simulink model "pwctrl"  (Simulink 7.8)
settings: Solver=FixedStepDiscrete  StartTime=0.0  StopTime=10  FixedStep=Ts  RelTol=1e-2
values from neighbouring files (symbols this model uses):
  EndStopThreshold = 15    [pwctrl_data.m]
  ObstacleThreshold = 1.2    [pwctrl_data.m]
undefined symbols (not defined in the file or in its folder): gcbh, rmidispblock
settings Model: RequirementInfo={'doors' '0000006a' '1' 'false' 'DOORS Surrogate Item' '' } %GIDa_dde32420_d5f5_4b5c_860d_5475e0ff803b  reqMgrSettings="100 S'doors','misc'{{S'surrogatepath','savemodel','savesurrogate','updateLinks','doorsLinks2sl','slLinks2Doors','purgeDoors','purgeSimulink','detaillevel','surrogateId','synctime'{{T\"/PowerWindow/pwctrl\",M[1],M[1],M[1],M[0],M[1],M[0],M[0],M[1],T\"0000006a\",T\"\"}},S'mode','pathStorage'{{T\"generic\",T\"modelRelative\"}}}}"  Creator=The MathWorks Inc.  LastModifiedBy=itoy  CovSaveName=covdatac  CovMetricSettings=dcmw  CovHTMLOptions=-aTS=1 -bRG=1 -bTC=1 -hTR=0 -nFC=0 -scm=1 -bcm=1 -xEv=0  CovCumulativeVarName=covCumulativeDataPwctrl  ExtModeAutoUpdateStatusClock=off
settings DataIOCC: SaveOutput=off  SaveTime=off  SignalLoggingName=sigsOut
settings OptimizationCC: InlineParams=on  InlineInvariantSignals=on  InitFltsAndDblsToZero=on  OptimizeModelRefInitCode=on  LifeSpan=1
settings DebuggingCC: SignalInfNanChecking=error  SaveWithParameterizedLinksMsg=none  CheckExecutionContextPreStartOutputMsg=on  CheckExecutionContextRuntimeOutputMsg=on  SolverPrmCheckMsg=none  MultiTaskDSMMsg=warning  MultiTaskCondExecSysMsg=none  ParameterUnderflowMsg=error  ParameterPrecisionLossMsg=error  ParameterTunabilityLossMsg=error  FcnCallInpInsideContextMsg=Use local settings  UniqueDataStoreMsg=warning  BusObjectLabelMismatch=error  RootOutportRequireBusObject=error  BusNameAdapt=ErrorWithoutRepair  NonBusSignalsTreatedAsBus=error
settings HardwareCC: ProdHWDeviceType=Generic->Unspecified (assume 32-bit Generic)  TargetIntDivRoundTo=Zero  TargetEndianess=LittleEndian  TargetHWDeviceType=Generic->MATLAB Host Computer  ProdEqTarget=off
settings SFSimCC: SimParseCustomCode=off
settings RTWCC: SystemTargetFile=ert.tlc  GenCodeOnly=on  TemplateMakefile=ert_default_tmf  Description=Real-Time Workshop Embedded Coder  GenerateReport=on  ProcessScript=ert_make_rtw_hook  IncludeHyperlinkInReport=on  LaunchReport=on  IncludeERTFirstTime=on  GenerateTraceInfo=on  GenerateTraceReport=on  GenerateTraceReportSl=on  GenerateTraceReportSf=on  GenerateTraceReportEml=on  GenerateCodeMetricsReport=on
settings MATStruct: className=rtw.pil.Bullseye  argsAllComponents=[]  excludedModels=[]  includeReferencedModels=off  includeTopModel=on  enabled=off
settings CodeAppCC: IgnoreCustomStorageClasses=off  CustomSymbolStrFcn=$F$N$M  ReqsInCode=on
settings ERTTargetCC: MultiwordLength=2048  GenerateSampleERTMain=on  SupportAbsoluteTime=off  SupportComplex=off  InlinedParameterPlacement=NonHierarchical  ERTCustomFileTemplate=example_file_process.tlc  ConvertIfToSwitch=off  SuppressUnreachableDefaultCases=off
settings SimMechanicsCC: WarnOnRedundantConstraints=off  VisOnUpdateDiagram=on
settings ConfigComp: Description=Design Verifier Custom Configuration Component  DVMaxProcessTime=600  DVDisplayUnsatisfiableObjectives=on  DVAutomaticStubbing=off  DVParametersConfigFileName=pwctrl_sldvparam.m  DVModelCoverageObjectives=MCDC  DVMaxTestCaseSteps=500  DVTestSuiteOptimization=CombinedObjectives (Nonlinear Extended)  DVIgnoreExistTestSatisfied=off  DVCoverageDataFile=C:\work\EXPO2010\demo\topmodelCov.cvt  DVSaveHarnessModel=on  DVSaveReport=on  DVDisplayResultsOnModel=on

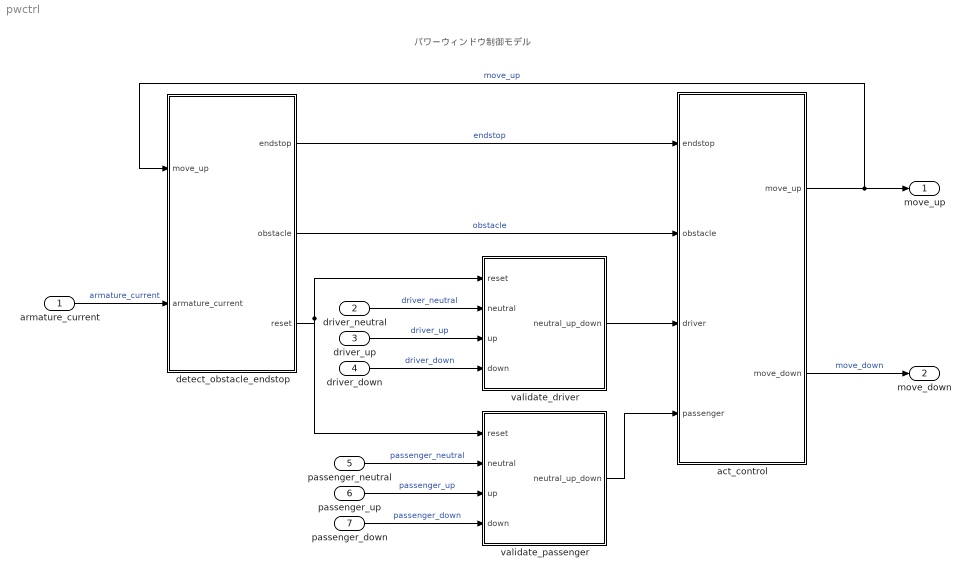
== system pwctrl ==
  note: パワーウィンドウ制御モデル
  armature_current : Inport  RequirementInfo={'other' 'powerwindowspecification.xlsx' '@Simulink_requirement_item_1' 'true' '電機子電流' '' } %GIDa_e1c18c69_aba9_407e_934a_76d29523162c  OutDataTypeStr=double  PortDimensions=1  Interpolate=off
  driver_neutral : Inport  RequirementInfo={'other' 'powerwindowspecification.xlsx' '@Simulink_requirement_item_2' 'true' '運転席ニュートラル命令' '' ; 'other' 'テスト01.docx' '@Simulink_requirement_item_1' 'true' 'テスト01' '' } %GIDa_63218ceb_c29f_4eb9_95a6_9012dd0a3532  Port=2  OutDataTypeStr=boolean  PortDimensions=1  Interpolate=off
  driver_up : Inport  RequirementInfo={'other' 'powerwindowspecification.xlsx' '@Simulink_requirement_item_3' 'true' '運転席アップ命令' '' } %GIDa_0b230fa1_5c49_495f_8d06_8dd23c30b7f9  Port=3  OutDataTypeStr=boolean  PortDimensions=1  Interpolate=off
  driver_down : Inport  RequirementInfo={'other' 'powerwindowspecification.xlsx' '@Simulink_requirement_item_4' 'true' '運転席ダウン命令' '' } %GIDa_6ce8d57e_d33e_47fb_aa6f_8cf7e75a9f12  Port=4  OutDataTypeStr=boolean  PortDimensions=1  Interpolate=off
  passenger_neutral : Inport  RequirementInfo={'other' 'powerwindowspecification.xlsx' '@Simulink_requirement_item_5' 'true' '助手席ニュートラル命令' '' } %GIDa_26eb5b41_6f4f_4623_9fef_cd17cf2cf6e8  Port=5  OutDataTypeStr=boolean  PortDimensions=1  Interpolate=off
  passenger_up : Inport  RequirementInfo={'other' 'powerwindowspecification.xlsx' '@Simulink_requirement_item_6' 'true' '助手席アップ命令' '' } %GIDa_f768338e_5d08_4c2e_8a73_e293dd283a19  Port=6  OutDataTypeStr=boolean  PortDimensions=1  Interpolate=off
  passenger_down : Inport  RequirementInfo={'other' 'powerwindowspecification.xlsx' '@Simulink_requirement_item_7' 'true' '助手席ダウン命令' '' } %GIDa_640f9234_8c00_498e_835c_04d6c270f85b  Port=7  OutDataTypeStr=boolean  PortDimensions=1  Interpolate=off
  act_control : Stateflow chart  RequirementInfo="{}  %GIDa_ef77f4d8_d6ef_4c80_8fd6_c4e6f18a1482"  TreatAsAtomicUnit=on
  detect_obstacle_endstop : Subsystem  RequirementInfo={'other' 'powerwindowspecification.xlsx' '@Simulink_requirement_item_75' 'true' 'PW02 障害物検知' '' ; 'other' 'powerwindowspecification.xlsx' '@Simulink_requirement_item_76' 'true' 'PW01-6' '' } %GIDa_a872e992_2f76_4f1e_be0d_48f835553ea8  TreatAsAtomicUnit=on
  validate_driver : Subsystem  RequirementInfo={'other' 'powerwindowspecification.xlsx' '@Simulink_requirement_item_74' 'true' 'PW01-1' '' ; 'other' 'powerwindowspecification.xlsx' '@Simulink_requirement_item_11' 'true' 'PW01-2' '' ; 'other' 'powerwindowspecification.xlsx' '@Simulink_requirement_item_12' 'true' 'PW01-3' '' } %GIDa_50d6339c_d923_4cb4_be9a_59dfda00bcf8  TreatAsAtomicUnit=on
  validate_passenger : Subsystem  RequirementInfo={'other' 'powerwindowspecification.xlsx' '@Simulink_requirement_item_13' 'true' 'PW01-4' '' ; 'other' 'powerwindowspecification.xlsx' '@Simulink_requirement_item_14' 'true' 'PW01-5' '' ; 'other' 'powerwindowspecification.xlsx' '@Simulink_requirement_item_15' 'true' 'PW01-6' '' } %GIDa_266d8f5a_6cdb_435d_b6a4_e11a48d16765  TreatAsAtomicUnit=on
  move_up : Outport  RequirementInfo={'other' 'powerwindowspecification.xlsx' '@Simulink_requirement_item_8' 'true' 'アップ指示' '' } %GIDa_af57c1a9_bee2_4bf2_aa23_d9548663e543  OutDataTypeStr=boolean
  move_down : Outport  RequirementInfo={'other' 'powerwindowspecification.xlsx' '@Simulink_requirement_item_9' 'true' 'ダウン指示' '' } %GIDa_5b47727d_3f56_4ff6_a9b6_2b328d3a62d1  Port=2  OutDataTypeStr=boolean
  wires:
  validate_passenger/1(neutral_up_down) -> act_control/4(passenger)
  validate_driver/1(neutral_up_down) -> act_control/3(driver)
  passenger_down/1 -> validate_passenger/4(down)  "passenger_down"
  passenger_up/1 -> validate_passenger/3(up)  "passenger_up"
  passenger_neutral/1 -> validate_passenger/2(neutral)  "passenger_neutral"
  driver_down/1 -> validate_driver/4(down)  "driver_down"
  driver_up/1 -> validate_driver/3(up)  "driver_up"
  driver_neutral/1 -> validate_driver/2(neutral)  "driver_neutral"
  act_control/2(move_down) -> move_down/1  "move_down"
  act_control/1(move_up) -> move_up/1, detect_obstacle_endstop/1(move_up)  "move_up"
  armature_current/1 -> detect_obstacle_endstop/2(armature_current)  "armature_current"
  detect_obstacle_endstop/3(reset) -> validate_driver/1(reset), validate_passenger/1(reset)
  detect_obstacle_endstop/1(endstop) -> act_control/1(endstop)  "endstop"
  detect_obstacle_endstop/2(obstacle) -> act_control/2(obstacle)  "obstacle"

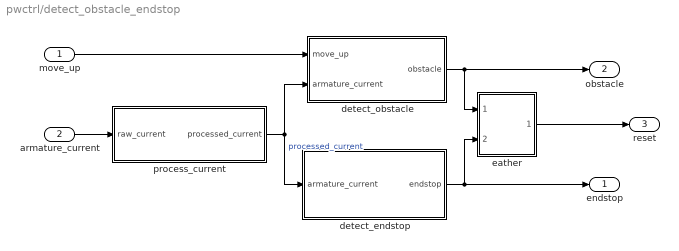
== system pwctrl/detect_obstacle_endstop ==
  move_up : Inport
  armature_current : Inport  Port=2
  detect_endstop : Subsystem  RequirementInfo={'other' 'powerwindowspecification.xlsx' '@Simulink_requirement_item_41' 'true' 'PW03-1' '' } %GIDa_aaa80572_f933_4bbe_b37f_c57c83952132
  detect_obstacle : Subsystem  RequirementInfo={'other' 'powerwindowspecification.xlsx' '@Simulink_requirement_item_33' 'true' 'PW02-1' '' } %GIDa_e14b3a63_7ae7_416e_9be9_c6135a02f311
  eather : Subsystem
  process_current : Subsystem  RequirementInfo={'other' 'powerwindowspecification.xlsx' '@Simulink_requirement_item_32' 'true' 'PW02-1' '' ; 'other' 'powerwindowspecification.xlsx' '@Simulink_requirement_item_40' 'true' 'PW03-1' '' } %GIDa_54e86e3e_ccc8_4b41_a5c1_edc4e8429aa2
  endstop : Outport
  obstacle : Outport  Port=2
  reset : Outport  Port=3
  wires:
  process_current/1(processed_current) -> detect_endstop/1(armature_current), detect_obstacle/2(armature_current)  "processed_current"
  move_up/1 -> detect_obstacle/1(move_up)
  eather/1(reset) -> reset/1
  detect_endstop/1(endstop) -> eather/2(endstop), endstop/1
  detect_obstacle/1(obstacle) -> obstacle/1, eather/1(obstacle)
  armature_current/1 -> process_current/1(raw_current)

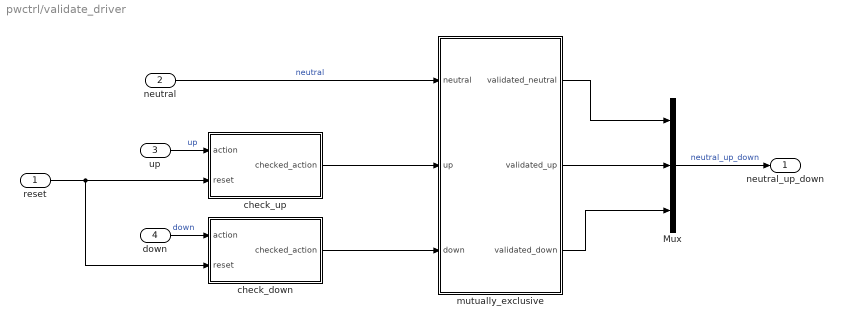
== system pwctrl/validate_driver ==
  reset : Inport
  neutral : Inport  Port=2
  up : Inport  Port=3
  down : Inport  Port=4
  Mux : Mux  Inputs=3
  check_down : Subsystem  RequirementInfo={'other' 'powerwindowspecification.xlsx' '@Simulink_requirement_item_55' 'true' 'PW02-4' '' ; 'other' 'powerwindowspecification.xlsx' '@Simulink_requirement_item_48' 'true' 'PW03-3' '' } %GIDa_8600958e_cd26_4390_bd74_0e0e2b2911b6
  check_up : Subsystem  RequirementInfo={'other' 'powerwindowspecification.xlsx' '@Simulink_requirement_item_54' 'true' 'PW02-4' '' ; 'other' 'powerwindowspecification.xlsx' '@Simulink_requirement_item_47' 'true' 'PW03-3' '' } %GIDa_854a0f09_eb00_4639_b606_a3908bff6a10
  mutually_exclusive : Subsystem  RequirementInfo={'other' 'powerwindowspecification.xlsx' '@Simulink_requirement_item_26' 'true' 'PW01-2-3' '' ; 'other' 'powerwindowspecification.xlsx' '@Simulink_requirement_item_29' 'true' 'PW01-1-3' '' } %GIDa_ad342d9f_5cab_43fb_a439_1578864a89a4
  neutral_up_down : Outport
  wires:
  Mux/1 -> neutral_up_down/1  "neutral_up_down"
  reset/1 -> check_down/2(reset), check_up/2(reset)
  check_up/1(checked_action) -> mutually_exclusive/2(up)
  neutral/1 -> mutually_exclusive/1(neutral)  "neutral"
  up/1 -> check_up/1(action)  "up"
  down/1 -> check_down/1(action)  "down"
  mutually_exclusive/1(validated_neutral) -> Mux/1
  mutually_exclusive/2(validated_up) -> Mux/2
  mutually_exclusive/3(validated_down) -> Mux/3
  check_down/1(checked_action) -> mutually_exclusive/3(down)

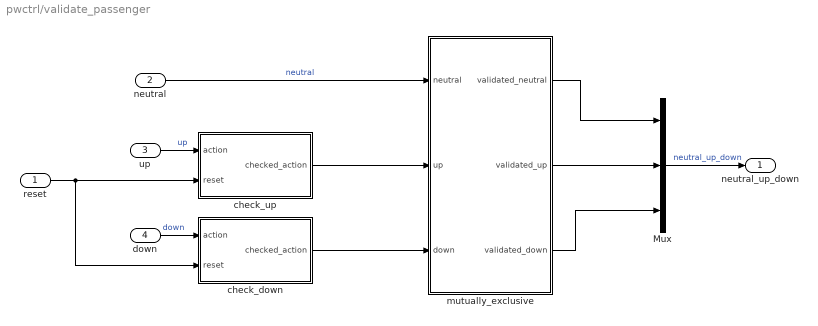
== system pwctrl/validate_passenger ==
  reset : Inport
  neutral : Inport  Port=2
  up : Inport  Port=3
  down : Inport  Port=4
  Mux : Mux  Inputs=3
  check_down : Subsystem  RequirementInfo={'other' 'powerwindowspecification.xlsx' '@Simulink_requirement_item_53' 'true' 'PW02-4' '' ; 'other' 'powerwindowspecification.xlsx' '@Simulink_requirement_item_50' 'true' 'PW03-3' '' } %GIDa_be4e89e9_75a8_4fb1_9b06_a19403e0c6cf
  check_up : Subsystem  RequirementInfo={'other' 'powerwindowspecification.xlsx' '@Simulink_requirement_item_52' 'true' 'PW02-4' '' ; 'other' 'powerwindowspecification.xlsx' '@Simulink_requirement_item_49' 'true' 'PW03-3' '' } %GIDa_c1637765_e427_4142_80f6_8167853f7876
  mutually_exclusive : Subsystem  RequirementInfo={'other' 'powerwindowspecification.xlsx' '@Simulink_requirement_item_28' 'true' 'PW01-5-3' '' ; 'other' 'powerwindowspecification.xlsx' '@Simulink_requirement_item_31' 'true' 'PW01-4-3' '' } %GIDa_ef85c54d_3e64_41b7_8079_161e00ee5cdb
  neutral_up_down : Outport
  wires:
  check_down/1(checked_action) -> mutually_exclusive/3(down)
  mutually_exclusive/3(validated_down) -> Mux/3
  mutually_exclusive/2(validated_up) -> Mux/2
  mutually_exclusive/1(validated_neutral) -> Mux/1
  down/1 -> check_down/1(action)  "down"
  up/1 -> check_up/1(action)  "up"
  neutral/1 -> mutually_exclusive/1(neutral)  "neutral"
  check_up/1(checked_action) -> mutually_exclusive/2(up)
  reset/1 -> check_up/2(reset), check_down/2(reset)
  Mux/1 -> neutral_up_down/1  "neutral_up_down"

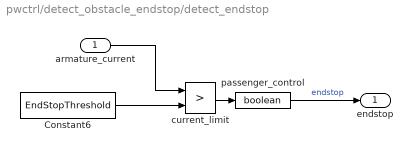
== system pwctrl/detect_obstacle_endstop/detect_endstop ==
  armature_current : Inport
  Constant6 : Constant  Value=EndStopThreshold  OutDataTypeStr=Inherit: Inherit via back propagation  SampleTime=Inf
  current_limit : RelationalOperator  Operator=>  InputSameDT=on
  passenger_control : DataTypeConversion  OutDataTypeStr=boolean  SaturateOnIntegerOverflow=on
  endstop : Outport
  wires:
  Constant6/1 -> current_limit/2
  armature_current/1 -> current_limit/1
  current_limit/1 -> passenger_control/1
  passenger_control/1 -> endstop/1  "endstop"

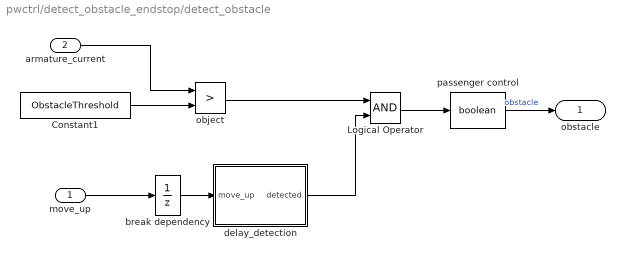
== system pwctrl/detect_obstacle_endstop/detect_obstacle ==
  move_up : Inport
  armature_current : Inport  Port=2
  Constant1 : Constant  Value=ObstacleThreshold
  Logical Operator : Logic  AllPortsSameDT=off  OutDataTypeStr=boolean
  break dependency : UnitDelay  SampleTime=-1
  delay_detection : Stateflow chart  TreatAsAtomicUnit=on
  object : RelationalOperator  Operator=>  InputSameDT=on
  passenger control : DataTypeConversion  OutDataTypeStr=boolean  SaturateOnIntegerOverflow=on
  obstacle : Outport
  wires:
  Constant1/1 -> object/2
  object/1 -> Logical Operator/1
  delay_detection/1(detected) -> Logical Operator/2
  armature_current/1 -> object/1
  move_up/1 -> break dependency/1
  Logical Operator/1 -> passenger control/1
  break dependency/1 -> delay_detection/1(move_up)
  passenger control/1 -> obstacle/1  "obstacle"

== system pwctrl/detect_obstacle_endstop/eather ==
  obstacle : Inport
  endstop : Inport  Port=2
  either : Logic  Operator=OR
  reset : Outport
  wires:
  obstacle/1 -> either/1
  endstop/1 -> either/2
  either/1 -> reset/1  "reset"

== system pwctrl/detect_obstacle_endstop/process_current ==
  raw_current : Inport
  Abs : Abs  SaturateOnIntegerOverflow=on
  processed_current : Outport
  wires:
  Abs/1 -> processed_current/1
  raw_current/1 -> Abs/1

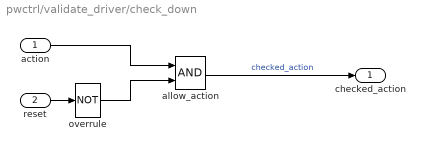
== system pwctrl/validate_driver/check_down ==
  action : Inport
  reset : Inport  Port=2
  allow_action : Logic
  overrule : Logic  Operator=NOT
  checked_action : Outport
  wires:
  reset/1 -> overrule/1
  allow_action/1 -> checked_action/1  "checked_action"
  action/1 -> allow_action/1
  overrule/1 -> allow_action/2

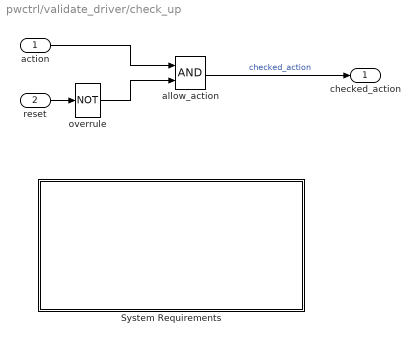
== system pwctrl/validate_driver/check_up ==
  action : Inport
  reset : Inport  Port=2
  System Requirements : Subsystem  LoadFcn=rmidispblock('load',gcbh)  mask(System Requirements){id=SystemReq, title=System Requirements}
      mask prompts: title "Block Title"
      mask help: Lists the requirements for the current model.
      mask init:
      | id = 'SystemReq';
      | [w,h] = rmidispblock('display',gcbh);
      settings: CopyFcn=rmidispblock('create',gcbh)  DeleteFcn=rmidispblock('delete',gcbh)  ModelCloseFcn=rmidispblock('close',gcbh)  PreSaveFcn=rmidispblock('close',gcbh)  PostSaveFcn=rmidispblock('open',gcbh)  OpenFcn=rmidispblock('open',gcbh)  MoveFcn=rmidispblock('move',gcbh)
      mask Help: web(slvnvhelp)
      mask Display: text(w/2,h-4,rmidispblock('title',gcbh),'horizontalAlignment','center','verticalAlignment','top')
  allow_action : Logic
  overrule : Logic  Operator=NOT
  checked_action : Outport
  wires:
  overrule/1 -> allow_action/2
  action/1 -> allow_action/1
  allow_action/1 -> checked_action/1  "checked_action"
  reset/1 -> overrule/1

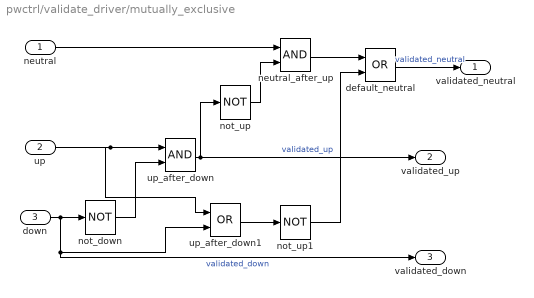
== system pwctrl/validate_driver/mutually_exclusive ==
  neutral : Inport
  up : Inport  Port=2
  down : Inport  Port=3
  default_neutral : Logic  Operator=OR
  neutral_after_up : Logic
  not_down : Logic  Operator=NOT
  not_up : Logic  Operator=NOT
  not_up1 : Logic  Operator=NOT
  up_after_down : Logic
  up_after_down1 : Logic  Operator=OR
  validated_neutral : Outport
  validated_up : Outport  Port=2
  validated_down : Outport  Port=3
  wires:
  not_down/1 -> up_after_down/2
  up_after_down/1 -> not_up/1, validated_up/1  "validated_up"
  not_up/1 -> neutral_after_up/2
  down/1 -> not_down/1, up_after_down1/2, validated_down/1  "validated_down"
  neutral/1 -> neutral_after_up/1
  up/1 -> up_after_down/1, up_after_down1/1
  up_after_down1/1 -> not_up1/1
  neutral_after_up/1 -> default_neutral/1
  default_neutral/1 -> validated_neutral/1  "validated_neutral"
  not_up1/1 -> default_neutral/2

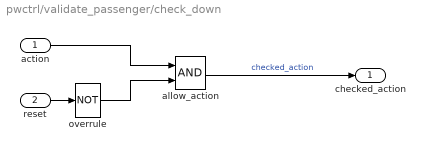
== system pwctrl/validate_passenger/check_down ==
  action : Inport
  reset : Inport  Port=2
  allow_action : Logic
  overrule : Logic  Operator=NOT
  checked_action : Outport
  wires:
  overrule/1 -> allow_action/2
  action/1 -> allow_action/1
  allow_action/1 -> checked_action/1  "checked_action"
  reset/1 -> overrule/1

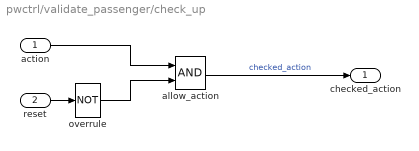
== system pwctrl/validate_passenger/check_up ==
  action : Inport
  reset : Inport  Port=2
  allow_action : Logic
  overrule : Logic  Operator=NOT
  checked_action : Outport
  wires:
  reset/1 -> overrule/1
  allow_action/1 -> checked_action/1  "checked_action"
  action/1 -> allow_action/1
  overrule/1 -> allow_action/2

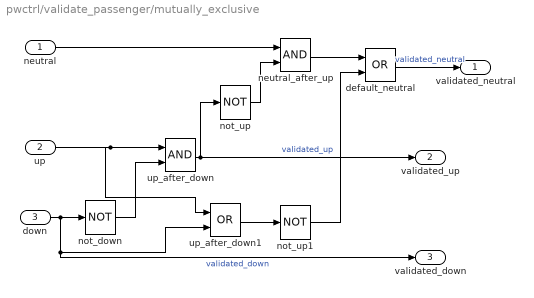
== system pwctrl/validate_passenger/mutually_exclusive ==
  neutral : Inport
  up : Inport  Port=2
  down : Inport  Port=3
  default_neutral : Logic  Operator=OR
  neutral_after_up : Logic
  not_down : Logic  Operator=NOT
  not_up : Logic  Operator=NOT
  not_up1 : Logic  Operator=NOT
  up_after_down : Logic
  up_after_down1 : Logic  Operator=OR
  validated_neutral : Outport
  validated_up : Outport  Port=2
  validated_down : Outport  Port=3
  wires:
  not_up1/1 -> default_neutral/2
  default_neutral/1 -> validated_neutral/1  "validated_neutral"
  neutral_after_up/1 -> default_neutral/1
  up_after_down1/1 -> not_up1/1
  up/1 -> up_after_down1/1, up_after_down/1
  neutral/1 -> neutral_after_up/1
  down/1 -> validated_down/1, up_after_down1/2, not_down/1  "validated_down"
  not_up/1 -> neutral_after_up/2
  up_after_down/1 -> validated_up/1, not_up/1  "validated_up"
  not_down/1 -> up_after_down/2

== system pwctrl/validate_driver/check_up/System Requirements ==
  Subsystem : Subsystem  mask{label=0, index=1}
      mask init:
      | label = rmidispblock('label',index);
      settings: OpenFcn=rmidispblock('openReq',gcbh);
      mask Display: text(0,0,label,'horizontalAlignment','left','verticalAlignment','bottom')

== system pwctrl/validate_driver/check_up/System Requirements/Subsystem ==

== stateflow chart act_control ==
  settings: executeAtInitialization=1
  state emergencyDown
    entry:
    move_up = 0;
    move_down = 1;
  state safe
    state driverUp
      entry:
      move_up = 1;
      exit:
      move_up = 0;
      state iniDriverUp
      state DriverUp
      state autoDriverUp
      iniDriverUp -> (junction 26) : [after(CountStep,tick)]
      (junction 26) -> DriverUp [order 2]
      (junction 26) -> autoDriverUp [order 1] : [driver[1]]
    state driverDown
      entry:
      move_down = 1;
      exit:
      move_down = 0;
      state iniDriverDown
      state DriverDown
      state autoDriverDown
      iniDriverDown -> (junction 25) : [after(CountStep,tick)]
      (junction 25) -> autoDriverDown [order 1] : [driver[1]]
      (junction 25) -> DriverDown [order 2]
    state driverNeutral
      entry:
      move_up = 0;
      move_down = 0;
      state passengerneutral
        entry:
        move_up = 0;
        move_down = 0;
      state passengerUp
        entry:
        move_up = 1;
        exit:
        move_up = 0;
        state iniPassengerUp
        state PassengerUp
        state autoPassengerUp
        (junction 24) -> PassengerUp [order 2]
        (junction 24) -> autoPassengerUp [order 1] : [passenger[1]]
        iniPassengerUp -> (junction 24) : [after(CountStep,tick)]
      state passengerDown
        entry:
        move_down = 1;
        exit:
        move_down = 0;
        state iniPassengerDown
        state passengerDown
        state autoPassengerDown
        (junction 23) -> autoPassengerDown [order 1] : [passenger[1]]
        iniPassengerDown -> (junction 23) : [after(CountStep,tick)]
        (junction 23) -> safe.driverNeutral.passengerDown.passengerDown [order 2]
      safe.driverNeutral.passengerDown.passengerDown -> passengerneutral : [passenger[1]]
      safe.driverNeutral.passengerDown -> passengerneutral [order 1] : [endstop]
      PassengerUp -> passengerneutral : [passenger[1]]
      passengerUp -> passengerneutral [order 1] : [endstop]
      passengerneutral -> iniPassengerDown [order 2] : [passenger[3]]
      passengerneutral -> iniPassengerUp [order 1] : [passenger[2]]
      safe.driverNeutral.passengerDown -> PassengerUp [order 2] : [passenger[2]]
      passengerUp -> safe.driverNeutral.passengerDown.passengerDown [order 2] : [passenger[3]]
      (default) -> passengerneutral
    driverNeutral -> iniDriverDown [order 2] : [driver[3]]
    driverUp -> DriverDown [order 2] : [driver[3]]
    driverDown -> DriverUp [order 2] : [driver[2]]
    driverNeutral -> iniDriverUp [order 1] : [driver[2]]
    DriverDown -> driverNeutral : [driver[1]]
    DriverUp -> driverNeutral : [driver[1]]
    driverDown -> driverNeutral [order 1] : [endstop]
    driverUp -> driverNeutral [order 1] : [endstop]
    (default) -> driverNeutral
  emergencyDown -> passengerneutral : [endstop | after(CountStep,tick)]
  safe -> emergencyDown : [obstacle]
  (default) -> safe
  data: move_up output boolean; move_down output boolean; endstop input boolean; obstacle input boolean; driver input boolean size=3; passenger input boolean size=3; CountStep parameter int16 =5

== stateflow chart detect_obstacle_endstop/detect_obstacle/delay_detection ==
  settings: sampleTime=Fs  executeAtInitialization=1
  state detect/
    en:
    detected = 1;
  state Off
    en:
    detected = 0;
  state hold
  (default) -> Off
  Off -> hold : [move_up]
  detect -> Off : [~move_up]
  hold -> detect [order 1] : [after(CountStep,tick)]
  hold -> Off [order 2] : [~move_up]
  data: move_up input boolean; CountStep parameter int16 =5; detected output boolean
